simulink model "glucagon"  (R2019a)
settings: Solver=VariableStepAuto  StartTime=0.0  StopTime=10.0  RelTol=1e-3
undefined symbols (not defined in the file): GHC_B, IHC_B
settings Model: Creator=rache  LastModifiedBy=rache
settings DataIOCC: ReturnWorkspaceOutputs=off
settings DebuggingCC: ArithmeticOperatorsInVariantConditions=warning

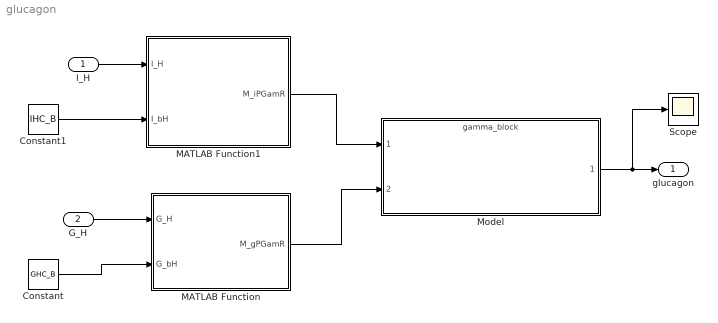
== system glucagon ==
  I_H : Inport
  G_H : Inport  Port=2
  Constant : Constant  Value=GHC_B
  Constant1 : Constant  Value=IHC_B
  MATLAB Function : MATLAB Function  TreatAsAtomicUnit=on
  MATLAB Function1 : MATLAB Function  TreatAsAtomicUnit=on
  Model : ModelReference  ModelNameDialog=gamma_block  SimulationMode=Normal  ModelReferenceVersion=1.4
  Scope : Scope
  glucagon : Outport
  wires:
  MATLAB Function1/1(M_iPGamR) -> Model/1
  MATLAB Function/1(M_gPGamR) -> Model/2
  I_H/1 -> MATLAB Function1/1(I_H)
  G_H/1 -> MATLAB Function/1(G_H)
  Model/1 -> Scope/1, glucagon/1
  Constant/1 -> MATLAB Function/2(G_bH)
  Constant1/1 -> MATLAB Function1/2(I_bH)

== matlab function glucagon/MATLAB Function1 ==
  data: I_H input; M_iPGamR output; I_bH input
function M_iPGamR = fcn(I_H, I_bH)

M_iPGamR = 2.93 - 2.09*(tanh(4.18*(I_H/I_bH - 0.62)));

== matlab function glucagon/MATLAB Function ==
  data: G_H input; M_gPGamR output; G_bH input
function M_gPGamR = fcn(G_H, G_bH)
M_gPGamR = 1.31 - 0.61*tanh(1.06*(G_H/G_bH - 0.47));
